simulink model "motorAdaptiveSim"  (R2016b)
settings: Solver=VariableStepAuto  StartTime=0.0  StopTime=100  RelTol=1e-3
undefined symbols (not defined in the file or in its folder): tf1
settings Model: Creator=julianleland  LastModifiedBy=julianleland

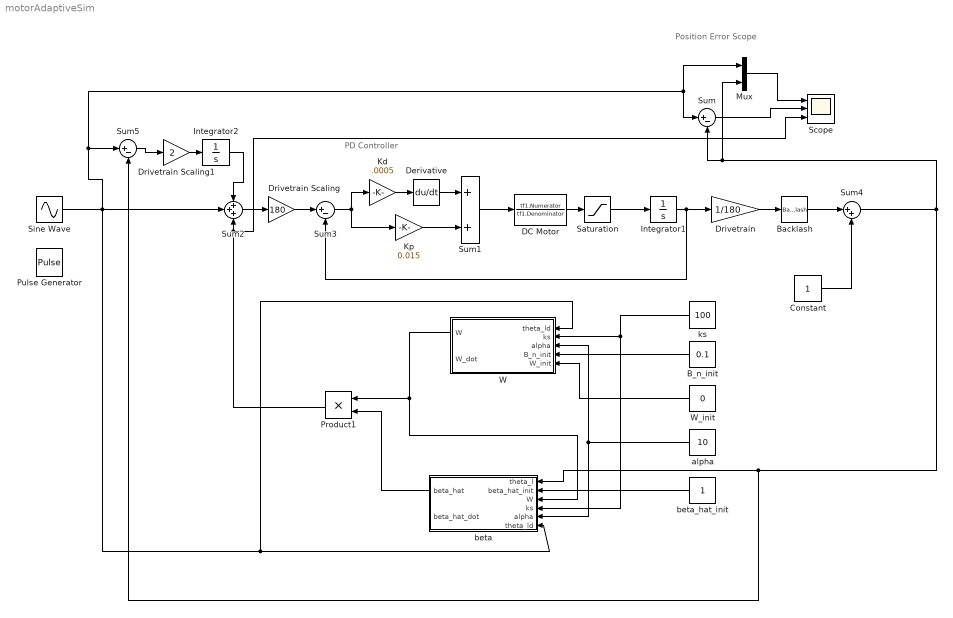
== system motorAdaptiveSim ==
  note: Position Error Scope
  note: PD Controller
  B_n_init : Constant  Value=0.1
  Backlash : Backlash  BacklashWidth=0.25
  Constant : Constant
  DC Motor : TransferFcn  Numerator=tf1.Numerator  Denominator=tf1.Denominator
  Derivative : Derivative
  Drivetrain : Gain  Gain=1/180
  Drivetrain Scaling : Gain  Gain=180
  Drivetrain Scaling1 : Gain  Gain=2
  Integrator1 : Integrator
  Integrator2 : Integrator  LimitOutput=on  UpperSaturationLimit=5  LowerSaturationLimit=-5
  Kd : Gain  Gain=.0005
  Kp : Gain  Gain=0.015
  Mux : Mux  Inputs=2
  Product1 : Product
  Pulse Generator : DiscretePulseGenerator  PulseType=Time based  Period=10  PulseWidth=50  PhaseDelay=0.5
  Saturation : Saturate  UpperLimit=460  LowerLimit=-460
  Scope : Scope  NumInputPorts=3
  Sine Wave : Sin  Amplitude=2  SampleTime=0
  Sum : Sum  Inputs=|+-
  Sum1 : Sum
  Sum2 : Sum  Inputs=+++
  Sum3 : Sum  Inputs=|+-
  Sum4 : Sum  Inputs=|++
  Sum5 : Sum  Inputs=|+-
  W : Subsystem
  W_init : Constant  Value=0
  alpha : Constant  Value=10
  beta : Subsystem
  beta_hat_init : Constant
  ks : Constant  Value=100
  wires:
  DC Motor/1 -> Saturation/1
  Integrator1/1 -> Sum3/2, Drivetrain/1
  Kp/1 -> Sum1/2
  Kd/1 -> Derivative/1
  Saturation/1 -> Integrator1/1
  Sum2/1 -> Drivetrain Scaling/1
  ks/1 -> beta/4(ks), W/2(ks)
  alpha/1 -> beta/5(alpha), W/3(alpha)
  B_n_init/1 -> W/4(B_n_init)
  W_init/1 -> W/5(W_init)
  W/1(W) -> beta/3(W), Product1/1
  beta_hat_init/1 -> beta/2(beta_hat_init)
  beta/1(beta_hat) -> Product1/2
  Drivetrain/1 -> Backlash/1
  Sum1/1 -> DC Motor/1
  Derivative/1 -> Sum1/1
  Sum3/1 -> Kd/1, Kp/1
  Drivetrain Scaling/1 -> Sum3/1
  Mux/1 -> Scope/1
  Sum/1 -> Scope/2
  Sum4/1 -> Mux/2, Sum/2, Sum5/2, beta/1(theta_l)
  Product1/1 -> Sum2/3, Scope/3
  Sine Wave/1 -> Sum2/2, Sum5/1, Mux/1, Sum/1, W/1(theta_ld), beta/6(theta_ld)
  Backlash/1 -> Sum4/1
  Constant/1 -> Sum4/2
  Sum5/1 -> Drivetrain Scaling1/1
  Drivetrain Scaling1/1 -> Integrator2/1
  Integrator2/1 -> Sum2/1

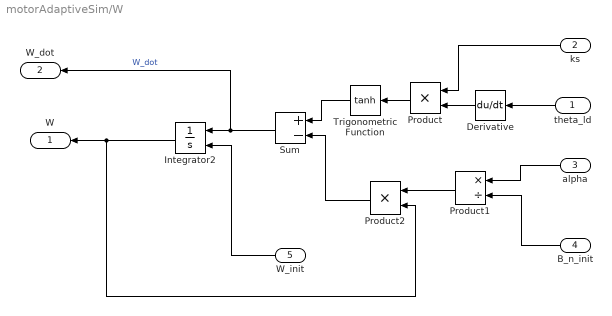
== system motorAdaptiveSim/W ==
  theta_ld : Inport
  ks : Inport  Port=2
  alpha : Inport  Port=3
  B_n_init : Inport  Port=4
  W_init : Inport  Port=5
  Derivative : Derivative
  Integrator2 : Integrator  InitialConditionSource=external
  Product : Product
  Product1 : Product  Inputs=*/
  Product2 : Product
  Sum : Sum  Inputs=+-
  Trigonometric Function : Trigonometry  Operator=tanh
  W : Outport
  W_dot : Outport  Port=2
  wires:
  Product2/1 -> Sum/2
  W_init/1 -> Integrator2/2
  Sum/1 -> Integrator2/1, W_dot/1  "W_dot"
  Trigonometric Function/1 -> Sum/1
  theta_ld/1 -> Derivative/1
  Product/1 -> Trigonometric Function/1
  Product1/1 -> Product2/1
  B_n_init/1 -> Product1/2
  alpha/1 -> Product1/1
  ks/1 -> Product/1
  Derivative/1 -> Product/2
  Integrator2/1 -> W/1, Product2/2

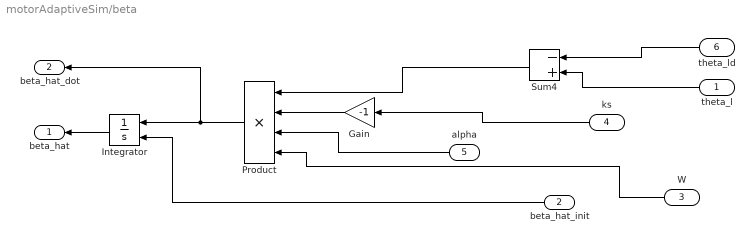
== system motorAdaptiveSim/beta ==
  theta_l : Inport
  beta_hat_init : Inport  Port=2
  W : Inport  Port=3
  ks : Inport  Port=4
  alpha : Inport  Port=5
  theta_ld : Inport  Port=6
  Gain : Gain  Gain=-1
  Integrator : Integrator  InitialConditionSource=external
  Product : Product  Inputs=****
  Sum4 : Sum  Inputs=-+
  beta_hat : Outport
  beta_hat_dot : Outport  Port=2
  wires:
  beta_hat_init/1 -> Integrator/2
  Integrator/1 -> beta_hat/1
  ks/1 -> Gain/1
  theta_ld/1 -> Sum4/1
  theta_l/1 -> Sum4/2
  alpha/1 -> Product/3
  W/1 -> Product/4
  Gain/1 -> Product/2
  Product/1 -> beta_hat_dot/1, Integrator/1
  Sum4/1 -> Product/1
